simulink model "schenario_1_input"  (R2019a)
settings: Solver=ode45  StartTime=0.0  StopTime=30  RelTol=1e-3  EnableMultiTasking=on
undefined symbols (not defined in the file): Omega_d_max
settings Model: Creator=Stelios  LastModifiedBy=Thanasis Charisoudis
settings DataIOCC: LimitDataPoints=on  SaveFormat=Array  InspectSignalLogs=on  ReturnWorkspaceOutputs=off
settings OptimizationCC: LifeSpan=inf
settings DebuggingCC: SFUnexpectedBacktrackingDiag=warning  SFNoUnconditionalDefaultTransitionDiag=warning  SFExecutionAtInitializationDiag=none  ArithmeticOperatorsInVariantConditions=warning
settings HardwareCC: ProdBitPerPointer=32  ProdBitPerSizeT=32  ProdBitPerPtrDiffT=32  ProdLargestAtomicFloat=None  ProdIntDivRoundTo=Undefined  ProdEndianess=Unspecified  ProdWordSize=32  ProdHWDeviceType=32-bit Generic
settings ModelReferenceCC: PropagateSignalLabelsOutOfModel=off
settings SFSimCC: SimUseLocalCustomCode=off
settings RTWCC: RTWUseLocalCustomCode=off
settings CodeAppCC: StateflowObjectComments=on
settings GRTTargetCC: TargetLangStandard=C89/C90 (ANSI)  GeneratePreprocessorConditionals=Disable all
settings ConfigComp: CovMetricSettings=dw  CovHtmlReporting=on  CovSaveCumulativeToWorkspaceVar=on  CovSaveSingleToWorkspaceVar=on  CovExternalEMLEnable=off

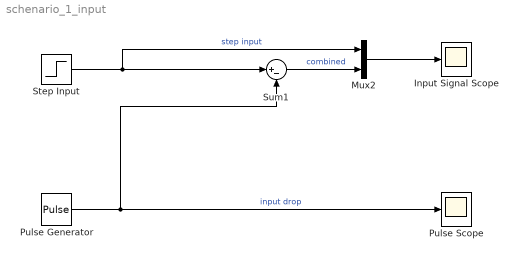
== system schenario_1_input ==
  Input Signal Scope : Scope
  Mux2 : Mux  Inputs=2
  Pulse Generator : DiscretePulseGenerator  PulseType=Time based  Amplitude=70  Period=50  PulseWidth=20  PhaseDelay=-35
  Pulse Scope : Scope
  "Step Input " : Step  Time=0  After=Omega_d_max  SampleTime=0.1
  Sum1 : Sum  Inputs=|+-  SaturateOnIntegerOverflow=on
  wires:
  "Step Input "/1 -> Mux2/1, Sum1/1  "step input"
  Sum1/1 -> Mux2/2  "combined"
  Pulse Generator/1 -> Sum1/2, Pulse Scope/1  "input drop"
  Mux2/1 -> Input Signal Scope/1
